simulink model "tabom"  (Simulink 8.4)
settings: Solver=ode45  StartTime=0.0  StopTime=20  RelTol=1e-3
undefined symbols (not defined in the file or in its folder): A, b, c, K, L
settings Model: Creator=Alunos  LastModifiedBy=Pedro
settings OptimizationCC: ExpressionDepthLimit=128  InitFltsAndDblsToZero=on
settings DebuggingCC: SaveWithParameterizedLinksMsg=none  SignalResolutionControl=TryResolveAllWithWarning  StateNameClashWarn=none
settings GRTTargetCC: TargetFcnLib=ansi_tfl_tmw.mat

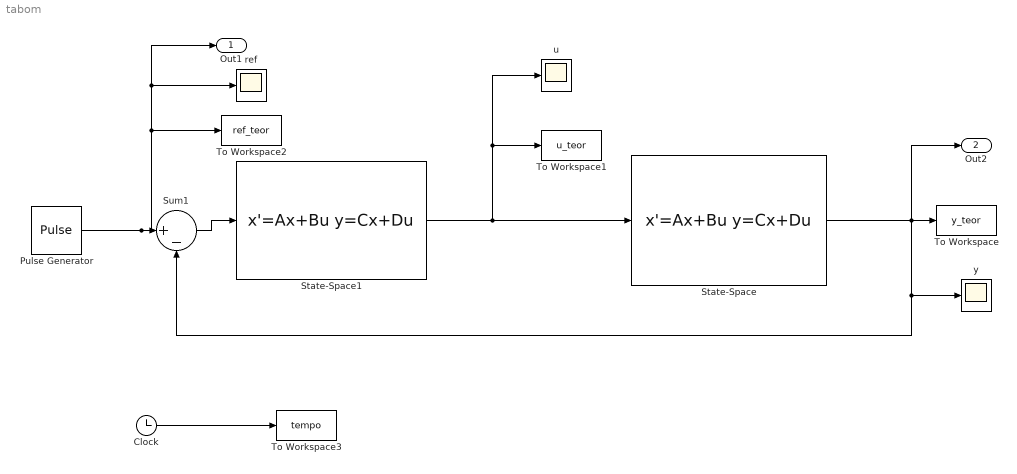
== system tabom ==
  Clock : Clock
  Pulse Generator : DiscretePulseGenerator  PulseType=Time based  Amplitude=.5  Period=5  PulseWidth=50
  State-Space : StateSpace  A=A  B=b  C=c  D=0  X0=0
  State-Space1 : StateSpace  A=A-b*K-L*c  B=-L  C=-K  D=0  X0=0
  Sum1 : Sum  Inputs=|+-
  To Workspace : ToWorkspace  VariableName=y_teor  SampleTime=-1
  To Workspace1 : ToWorkspace  VariableName=u_teor  SampleTime=-1
  To Workspace2 : ToWorkspace  VariableName=ref_teor  SampleTime=-1
  To Workspace3 : ToWorkspace  VariableName=tempo  SampleTime=-1
  ref : Scope
  u : Scope
      settings: SaveName=ScopeData2
  y : Scope
  Out1 : Outport
  Out2 : Outport  Port=2
  wires:
  State-Space/1 -> To Workspace/1, y/1, Sum1/2, Out2/1
  State-Space1/1 -> State-Space/1, To Workspace1/1, u/1
  Pulse Generator/1 -> Sum1/1, To Workspace2/1, ref/1, Out1/1
  Sum1/1 -> State-Space1/1
  Clock/1 -> To Workspace3/1
